simulink model "Dan_model2a"  (Simulink 7.8)
settings: Solver=ode45  StartTime=0.0  StopTime=10.0  RelTol=1e-3
values from neighbouring files (symbols this model uses):
  a = avect(i)    [ps7-p1.m]    (also in ps7-task2.m = -1)
  shift = 30    [ps7-p1.m]
libraries: dsparch4 x1
settings Model: Creator=Dan  LastModifiedBy=Dan
settings DebuggingCC: InitInArrayFormatMsg=none

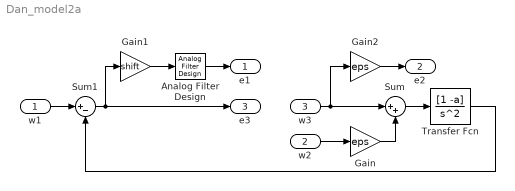
== system Dan_model2a ==
  w1 : Inport
  w2 : Inport  Port=2
  w3 : Inport  Port=3
  Analog Filter Design : dsparch4/Analog Filter Design  method=Butterworth  filttype=Lowpass  N=2  Wlo=passband  Whi=80  Rp=2  Rs=40
  Gain : Gain  Gain=eps
  Gain1 : Gain  Gain=shift
  Gain2 : Gain  Gain=eps
  Sum : Sum  Inputs=|++
  Sum1 : Sum  Inputs=|+-
  Transfer Fcn : TransferFcn  Numerator=[1 -a]  Denominator=[1 0 0]
  e1 : Outport
  e2 : Outport  Port=2
  e3 : Outport  Port=3
  wires:
  Sum/1 -> Transfer Fcn/1
  w2/1 -> Gain/1
  Sum1/1 -> Gain1/1, e3/1
  w1/1 -> Sum1/1
  Gain2/1 -> e2/1
  Transfer Fcn/1 -> Sum1/2
  Analog Filter Design/1 -> e1/1
  Gain1/1 -> Analog Filter Design/1
  w3/1 -> Gain2/1, Sum/1
  Gain/1 -> Sum/2
